simulink model "Gaussian_Principle"  (R2024b)
settings: Solver=FixedStepAuto  StartTime=0.0  StopTime=10.0  FixedStep=0.01  RelTol=1e-3
values from neighbouring files (symbols this model uses):
  Dr_m = 0.001    [Gaussian_Variable.m]
  P1_Pa = 16000    [Gaussian_Variable.m]
  p_kgpm3 = 1060    [Gaussian_Variable.m]
  pi_nd = 3.14    [Gaussian_Variable.m]
  Q_m3ps = 0.0000015    (= 1.5e-06)    [Gaussian_Variable.m]
  r0_m = 0.002    [Gaussian_Variable.m]
  sig_m = 0.0009    [Gaussian_Variable.m]
  x0_m = 0    [Gaussian_Variable.m]
  x_m = 0.001    [Gaussian_Variable.m]
settings Model: Creator=Stephon Woodson  LastModifiedBy=Stephon Woodson

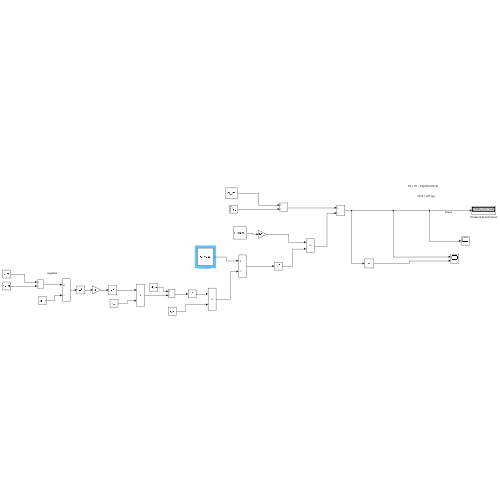
[thumbnail: Simulink's stored preview of the top-level diagram]
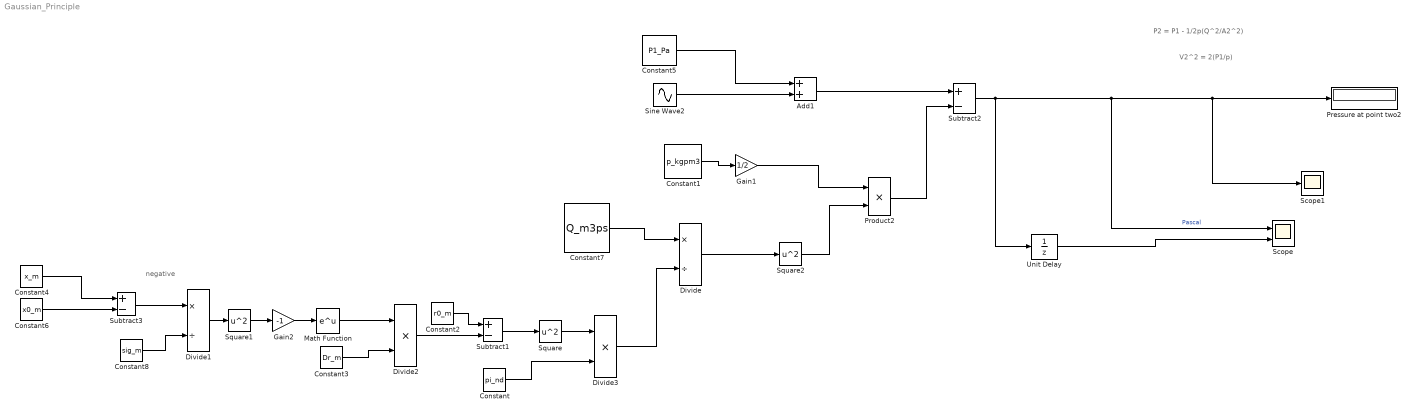
== system Gaussian_Principle ==
  note: negative
  note: P2 = P1 - 1/2p(Q^2/A2^2)
  note: V2^2 = 2(P1/p)
  Add1 : Sum
  Constant : Constant  Value=pi_nd
  Constant1 : Constant  Value=p_kgpm3
  Constant2 : Constant  Value=r0_m
  Constant3 : Constant  Value=Dr_m
  Constant4 : Constant  Value=x_m
  Constant5 : Constant  Value=P1_Pa
  Constant6 : Constant  Value=x0_m
  Constant7 : Constant  Value=Q_m3ps
  Constant8 : Constant  Value=sig_m
  Divide : Product  Inputs=*/
  Divide1 : Product  Inputs=*/
  Divide2 : Product  Inputs=**
  Divide3 : Product  Inputs=**
  Gain1 : Gain  Gain=1/2
  Gain2 : Gain  Gain=-1
  Math Function : Math
  Pressure at point two2 : Display
  Product2 : Product
  Scope : Scope  NumInputPorts=2
  Scope1 : Scope
  Sine Wave2 : Sin  SampleTime=0
  Square : Math  Operator=square
  Square1 : Math  Operator=square
  Square2 : Math  Operator=square
  Subtract1 : Sum  Inputs=+-
  Subtract2 : Sum  Inputs=+-
  Subtract3 : Sum  Inputs=+-
  Unit Delay : UnitDelay  InitialCondition=15985.82  SampleTime=-1  HasFrameUpgradeWarning=on
  wires:
  Gain1/1 -> Product2/1
  Square2/1 -> Product2/2
  Subtract2/1 -> Unit Delay/1, Scope/1, Scope1/1, Pressure at point two2/1  "Pascal"
  Divide/1 -> Square2/1
  Product2/1 -> Subtract2/2
  Add1/1 -> Subtract2/1
  Constant7/1 -> Divide/1
  Constant1/1 -> Gain1/1
  Constant5/1 -> Add1/1
  Sine Wave2/1 -> Add1/2
  Constant2/1 -> Subtract1/1
  Constant4/1 -> Subtract3/1
  Constant6/1 -> Subtract3/2
  Subtract3/1 -> Divide1/1
  Constant8/1 -> Divide1/2
  Divide1/1 -> Square1/1
  Square1/1 -> Gain2/1
  Gain2/1 -> Math Function/1
  Math Function/1 -> Divide2/1
  Divide3/1 -> Divide/2
  Constant3/1 -> Divide2/2
  Divide2/1 -> Subtract1/2
  Subtract1/1 -> Square/1
  Square/1 -> Divide3/1
  Constant/1 -> Divide3/2
  Unit Delay/1 -> Scope/2
